simulink model "bh_COMPONENT_car_sys"  (R2018a)
settings: Solver=ode45  StartTime=0.0  StopTime=20  FixedStep=0.001  RelTol=1e-5
undefined symbols (not defined in the file): Ke, mot_bR, mot_COM, veh
libraries: simulink_extras x3, simulink x2
settings Model: Creator=bhorton  LastModifiedBy=bhorton
settings SolverCC: ZeroCrossControl=EnableAll  ZeroCrossAlgorithm=Adaptive
settings DebuggingCC: SignalInfNanChecking=warning
settings ModelReferenceCC: ModelReferenceMinAlgLoopOccurrences=on

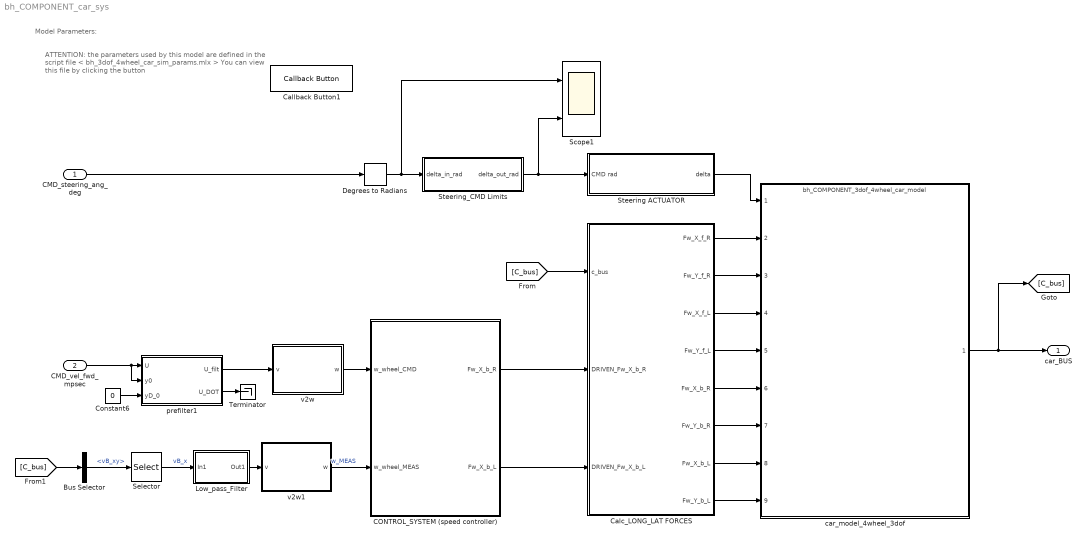
== system bh_COMPONENT_car_sys ==
  note: Model Parameters:
  note: ATTENTION:
      | the parameters used by this model are defined in the script file
      | < bh_3dof_4wheel_car_sim_params.mlx >
      |
      | You can view this file by clicking the button
  CMD_steering_ang_deg : Inport
  CMD_vel_fwd_mpsec : Inport  Port=2
  Bus Selector : BusSelector  OutputSignals=states_B.vB_xy
  CONTROL_SYSTEM (speed controller) : Subsystem  Variant=on  OverrideUsingVariant=Variant1
  Calc_LONG_LAT FORCES : Subsystem
  Callback Button1 : CallbackButton  WebBlockId=2544  ButtonText=view parameter file
      settings: ClickFcn=edit bh_3dof_4wheel_car_sim_params.mlx
  Constant6 : Constant  Value=0
  Degrees to Radians : simulink_extras/Transformations/Degrees to Radians
  Low_pass_Filter : Subsystem
  Scope1 : Scope  NumInputPorts=2
  Selector : Selector  InputPortWidth=2  IndexOptions=Index vector (dialog)  Indices=1  OutputSizes=1
  Steering ACTUATOR : Subsystem
  Steering_CMD Limits : Subsystem
  Terminator : Terminator
  car_model_4wheel_3dof : ModelReference  ModelNameDialog=bh_COMPONENT_3dof_4wheel_car_model.slx  SimulationMode=Normal  ModelReferenceVersion=1.187
  prefilter1 : Subsystem  mask(Derivative Estimation){wn=2*pi*5, p=1}
      mask prompts: wn "Natural frequency, wn (rad/sec)"; p "Damping ratio, p"
      mask help:
      | A simple derivative estimator using a 2nd order representation between input and output.
      |
      | The integrators use a discrete FORWARd Euler rule, and a sample time needs to be specified.
      mask init:
      | str1 = sprintf('wn = %.2f', wn);
      | str2 = sprintf('p  = %.2f', p);
      | %str3 = sprintf('dt = %.2f', dt);
      | %str = char(str1,str2,str3);
      | %str3 = sprintf('dt = %.2f', dt);
      | str = char(str1,str2);
      mask Display: disp(str)
  v2w : Subsystem  mask(v2w){r=veh.wheel.r}
      mask prompts: r "wheel radius (m)"
      mask help:
      | convert v into w
      | w = v/r
      mask Display: image(imread('bh_PIC_v2w.JPG'),'center')
  v2w1 : Subsystem  mask(v2w){r=veh.wheel.r}
      mask prompts: r "wheel radius (m)"
      mask help:
      | convert v into w
      | w = v/r
      mask Display: image(imread('bh_PIC_v2w.JPG'),'center')
  car_BUS : Outport  OutDataTypeStr=Bus: car_BUS
  wires:
  [C_bus] -> Calc_LONG_LAT FORCES/1(c_bus)
  Degrees to Radians/1 -> Scope1/1, Steering_CMD Limits/1(delta_in_rad)
  [C_bus] -> Bus Selector/1
  CMD_vel_fwd_mpsec/1 -> prefilter1/2(y0), prefilter1/1(U)
  Constant6/1 -> prefilter1/3(yD_0)
  CMD_steering_ang_deg/1 -> Degrees to Radians/1
  Steering_CMD Limits/1(delta_out_rad) -> Scope1/2, Steering ACTUATOR/1(CMD rad)
  car_model_4wheel_3dof/1 -> car_BUS/1, [C_bus]
  Steering ACTUATOR/1(delta) -> car_model_4wheel_3dof/1
  Calc_LONG_LAT FORCES/1(Fw_X_f_R) -> car_model_4wheel_3dof/2
  Calc_LONG_LAT FORCES/2(Fw_Y_f_R) -> car_model_4wheel_3dof/3
  Calc_LONG_LAT FORCES/3(Fw_X_f_L) -> car_model_4wheel_3dof/4
  Calc_LONG_LAT FORCES/4(Fw_Y_f_L) -> car_model_4wheel_3dof/5
  Calc_LONG_LAT FORCES/5(Fw_X_b_R) -> car_model_4wheel_3dof/6
  Calc_LONG_LAT FORCES/6(Fw_Y_b_R) -> car_model_4wheel_3dof/7
  Calc_LONG_LAT FORCES/7(Fw_X_b_L) -> car_model_4wheel_3dof/8
  Calc_LONG_LAT FORCES/8(Fw_Y_b_L) -> car_model_4wheel_3dof/9
  prefilter1/1(U_filt) -> v2w/1(v)
  Low_pass_Filter/1(Out1) -> v2w1/1(v)
  v2w/1(w) -> CONTROL_SYSTEM (speed controller)/1(w_wheel_CMD)
  v2w1/1(w) -> CONTROL_SYSTEM (speed controller)/2(w_wheel_MEAS)  "w_MEAS"
  CONTROL_SYSTEM (speed controller)/2(Fw_X_b_L) -> Calc_LONG_LAT FORCES/3(DRIVEN_Fw_X_b_L)
  CONTROL_SYSTEM (speed controller)/1(Fw_X_b_R) -> Calc_LONG_LAT FORCES/2(DRIVEN_Fw_X_b_R)
  Bus Selector/1 -> Selector/1  "<vB_xy>"
  Selector/1 -> Low_pass_Filter/1(In1)  "vB_x"
  prefilter1/2(U_DOT) -> Terminator/1

== system bh_COMPONENT_car_sys/CONTROL_SYSTEM (speed controller) ==
  note: 1) Add Subsystem or Model blocks as valid variant choices.
      | 2) You cannot connect blocks at this level. At simulation, connectivity is automatically
      | determined, based on the active variant and port name matching.
  w_wheel_CMD : Inport
  w_wheel_MEAS : Inport  Port=2
  DC_motor_simple_FRICT : Subsystem  VariantControl=Variant1
  IDEAL_FORCE_ACTUATOR_SYS : Subsystem  VariantControl=Variant3
  Fw_X_b_R : Outport
  Fw_X_b_L : Outport  Port=2

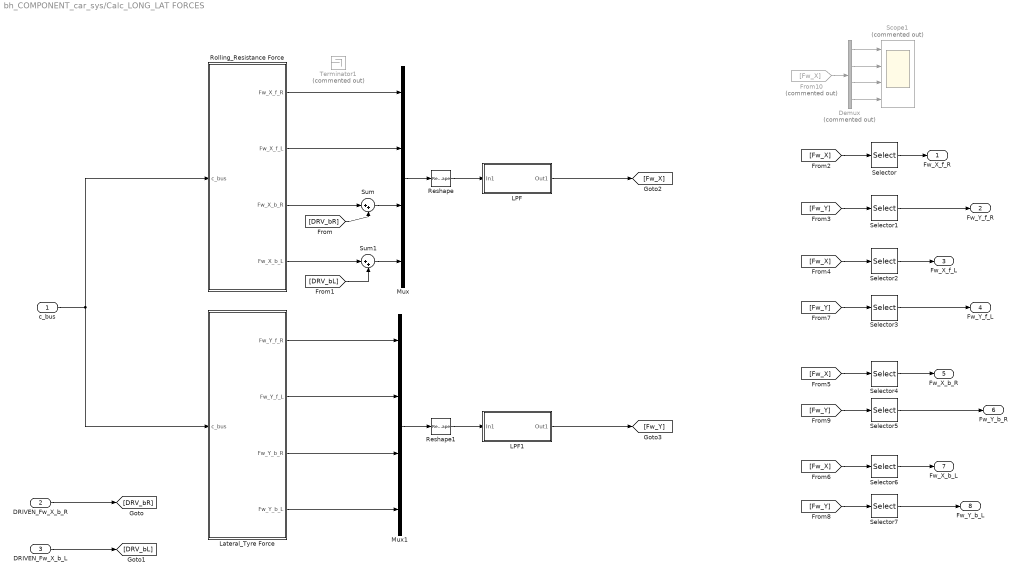
== system bh_COMPONENT_car_sys/Calc_LONG_LAT FORCES ==
  c_bus : Inport
  DRIVEN_Fw_X_b_R : Inport  Port=2
  DRIVEN_Fw_X_b_L : Inport  Port=3
  Demux : Demux  Commented=on
  From10 : From  Commented=on  GotoTag=Fw_X
  LPF : Subsystem
  LPF1 : Subsystem
  Lateral_Tyre Force : Subsystem
  Mux : Mux
  Mux1 : Mux
  Reshape : Reshape  OutputDimensionality=Column vector (2-D)
  Reshape1 : Reshape  OutputDimensionality=Column vector (2-D)
  Rolling_Resistance Force : Subsystem
  Scope1 : Scope  Commented=on  NumInputPorts=4
  Selector : Selector  InputPortWidth=4  IndexOptions=Index vector (dialog)  Indices=1  OutputSizes=1
  Selector1 : Selector  InputPortWidth=4  IndexOptions=Index vector (dialog)  Indices=1  OutputSizes=1
  Selector2 : Selector  InputPortWidth=4  IndexOptions=Index vector (dialog)  Indices=2  OutputSizes=1
  Selector3 : Selector  InputPortWidth=4  IndexOptions=Index vector (dialog)  Indices=2  OutputSizes=1
  Selector4 : Selector  InputPortWidth=4  IndexOptions=Index vector (dialog)  Indices=3  OutputSizes=1
  Selector5 : Selector  InputPortWidth=4  IndexOptions=Index vector (dialog)  Indices=3  OutputSizes=1
  Selector6 : Selector  InputPortWidth=4  IndexOptions=Index vector (dialog)  Indices=4  OutputSizes=1
  Selector7 : Selector  InputPortWidth=4  IndexOptions=Index vector (dialog)  Indices=4  OutputSizes=1
  Sum : Sum  Inputs=|++
  Sum1 : Sum  Inputs=|++
  Terminator1 : Terminator  Commented=on
  Fw_X_f_R : Outport
  Fw_Y_f_R : Outport  Port=2
  Fw_X_f_L : Outport  Port=3
  Fw_Y_f_L : Outport  Port=4
  Fw_X_b_R : Outport  Port=5
  Fw_Y_b_R : Outport  Port=6
  Fw_X_b_L : Outport  Port=7
  Fw_Y_b_L : Outport  Port=8
  wires:
  Selector/1 -> Fw_X_f_R/1
  Selector5/1 -> Fw_Y_b_R/1
  Selector7/1 -> Fw_Y_b_L/1
  Selector1/1 -> Fw_Y_f_R/1
  c_bus/1 -> Rolling_Resistance Force/1(c_bus), Lateral_Tyre Force/1(c_bus)
  DRIVEN_Fw_X_b_R/1 -> [DRV_bR]
  DRIVEN_Fw_X_b_L/1 -> [DRV_bL]
  Rolling_Resistance Force/2(Fw_X_f_L) -> Mux/2
  Rolling_Resistance Force/1(Fw_X_f_R) -> Mux/1
  Lateral_Tyre Force/1(Fw_Y_f_R) -> Mux1/1
  Lateral_Tyre Force/2(Fw_Y_f_L) -> Mux1/2
  Lateral_Tyre Force/3(Fw_Y_b_R) -> Mux1/3
  Lateral_Tyre Force/4(Fw_Y_b_L) -> Mux1/4
  Mux1/1 -> Reshape1/1
  Mux/1 -> Reshape/1
  [Fw_Y] -> Selector1/1
  [Fw_X] -> Selector/1
  Selector6/1 -> Fw_X_b_L/1
  Selector4/1 -> Fw_X_b_R/1
  Selector3/1 -> Fw_Y_f_L/1
  Selector2/1 -> Fw_X_f_L/1
  [Fw_Y] -> Selector7/1
  [Fw_X] -> Selector6/1
  [Fw_Y] -> Selector5/1
  [Fw_X] -> Selector4/1
  [Fw_Y] -> Selector3/1
  [Fw_X] -> Selector2/1
  Reshape/1 -> LPF/1(In1)
  LPF/1(Out1) -> [Fw_X]
  LPF1/1(Out1) -> [Fw_Y]
  Demux/1 -> Scope1/1
  Demux/2 -> Scope1/2
  Demux/3 -> Scope1/3
  Demux/4 -> Scope1/4
  From10/1 -> Demux/1
  Rolling_Resistance Force/3(Fw_X_b_R) -> Sum/1
  [DRV_bR] -> Sum/2
  Sum1/1 -> Mux/4
  Rolling_Resistance Force/4(Fw_X_b_L) -> Sum1/1
  [DRV_bL] -> Sum1/2
  Sum/1 -> Mux/3
  Reshape1/1 -> LPF1/1(In1)

== system bh_COMPONENT_car_sys/Low_pass_Filter ==
  In1 : Inport
  Constant2 : Constant  Value=0
  Terminator1 : Terminator
  prefilter2 : Subsystem  mask(Derivative Estimation){wn=2*pi*100, p=1}
      mask prompts: wn "Natural frequency, wn (rad/sec)"; p "Damping ratio, p"
      mask help:
      | A simple derivative estimator using a 2nd order representation between input and output.
      |
      | The integrators use a discrete FORWARd Euler rule, and a sample time needs to be specified.
      mask init:
      | str1 = sprintf('wn = %.2f', wn);
      | str2 = sprintf('p  = %.2f', p);
      | %str3 = sprintf('dt = %.2f', dt);
      | %str = char(str1,str2,str3);
      | %str3 = sprintf('dt = %.2f', dt);
      | str = char(str1,str2);
      mask Display: disp(str)
  Out1 : Outport
  wires:
  prefilter2/2(U_DOT) -> Terminator1/1
  In1/1 -> prefilter2/1(U)
  prefilter2/1(U_filt) -> Out1/1
  Constant2/1 -> prefilter2/3(yD_0), prefilter2/2(y0)

== system bh_COMPONENT_car_sys/Steering ACTUATOR ==
  CMD rad : Inport
  2nd_order_TF : Subsystem  mask(Derivative Estimation){wn=2*pi*10, p=1}
      mask prompts: wn "Natural frequency, wn (rad/sec)"; p "Damping ratio, p"
      mask help:
      | A simple derivative estimator using a 2nd order representation between input and output.
      |
      | The integrators use a discrete FORWARd Euler rule, and a sample time needs to be specified.
      mask init:
      | str1 = sprintf('wn = %.2f', wn);
      | str2 = sprintf('p  = %.2f', p);
      | %str3 = sprintf('dt = %.2f', dt);
      | %str = char(str1,str2,str3);
      | %str3 = sprintf('dt = %.2f', dt);
      | str = char(str1,str2);
      mask Display: disp(str)
  Constant2 : Constant  Value=0
  Terminator1 : Terminator
  delta : Outport
  wires:
  2nd_order_TF/2(U_DOT) -> Terminator1/1
  CMD rad/1 -> 2nd_order_TF/1(U)
  2nd_order_TF/1(U_filt) -> delta/1
  Constant2/1 -> 2nd_order_TF/3(yD_0), 2nd_order_TF/2(y0)

== system bh_COMPONENT_car_sys/Steering_CMD Limits ==
  note: Saturate on DEGREES
  delta_in_rad : Inport
  Degrees to Radians : simulink_extras/Transformations/Degrees to Radians
  Radians to Degrees : simulink_extras/Transformations/Radians to Degrees
  Saturation : Saturate  UpperLimit=veh.steering_delta_deg_max  LowerLimit=veh.steering_delta_deg_min
      settings: AttributesFormatString=|
      | MAX = %<UpperLimit>
      | MIN = %<LowerLimit>
  delta_out_rad : Outport
  wires:
  delta_in_rad/1 -> Radians to Degrees/1  "radians"
  Saturation/1 -> Degrees to Radians/1  "degrees"
  Radians to Degrees/1 -> Saturation/1  "degrees"
  Degrees to Radians/1 -> delta_out_rad/1  "radians"

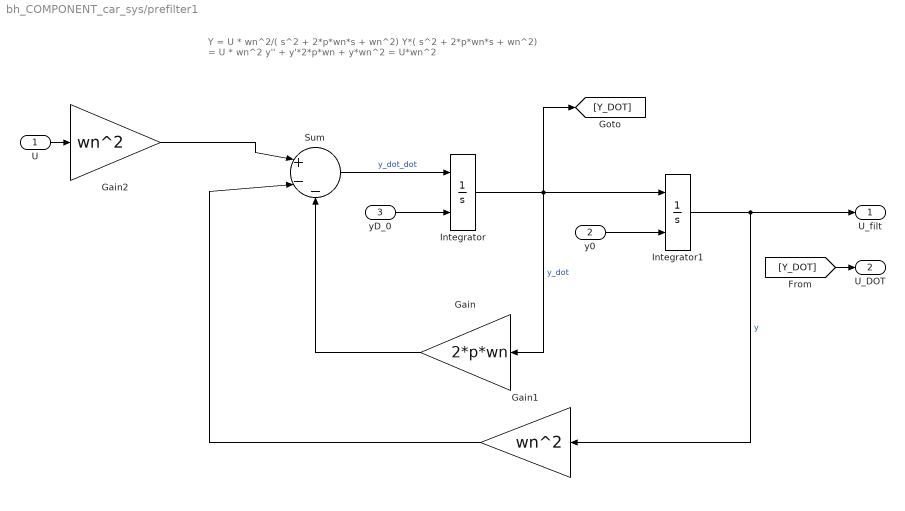
== system bh_COMPONENT_car_sys/prefilter1 ==
  note: Y = U *     wn^2/( s^2 + 2*p*wn*s + wn^2)
      | Y*( s^2 + 2*p*wn*s + wn^2) = U * wn^2
      |
      | y'' + y'*2*p*wn + y*wn^2 = U*wn^2
  U : Inport
  y0 : Inport  Port=2
  yD_0 : Inport  Port=3
  Gain : Gain  Gain=2*p*wn
  Gain1 : Gain  Gain=wn^2
  Gain2 : Gain  Gain=wn^2
  Integrator : Integrator  InitialConditionSource=external
  Integrator1 : Integrator  InitialConditionSource=external
  Sum : Sum  Inputs=|+--
  U_filt : Outport
  U_DOT : Outport  Port=2
  wires:
  Integrator/1 -> [Y_DOT], Gain/1, Integrator1/1  "y_dot"
  Sum/1 -> Integrator/1  "y_dot_dot"
  Integrator1/1 -> Gain1/1, U_filt/1  "y"
  U/1 -> Gain2/1
  Gain2/1 -> Sum/1
  Gain/1 -> Sum/3
  Gain1/1 -> Sum/2
  [Y_DOT] -> U_DOT/1
  yD_0/1 -> Integrator/2
  y0/1 -> Integrator1/2

== system bh_COMPONENT_car_sys/v2w ==
  note: w = v/r
  v : Inport
  Gain : Gain  Gain=1/r
  w : Outport
  wires:
  v/1 -> Gain/1
  Gain/1 -> w/1

== system bh_COMPONENT_car_sys/v2w1 ==
  note: w = v/r
  v : Inport
  Gain : Gain  Gain=1/r
  w : Outport
  wires:
  v/1 -> Gain/1
  Gain/1 -> w/1

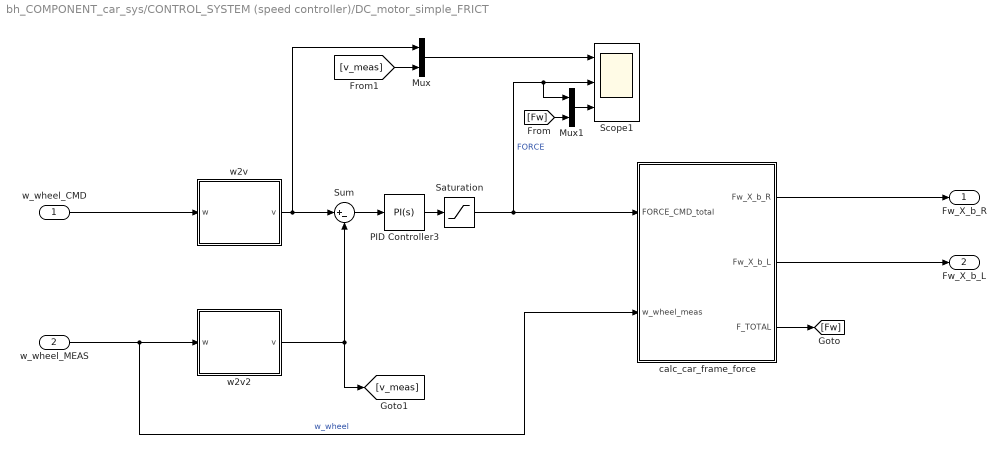
== system bh_COMPONENT_car_sys/CONTROL_SYSTEM (speed controller)/DC_motor_simple_FRICT ==
  w_wheel_CMD : Inport
  w_wheel_MEAS : Inport  Port=2
  Mux : Mux  Inputs=2
  Mux1 : Mux  Inputs=2
  PID Controller3 : simulink/Continuous/PID Controller  Controller=PI  TimeDomain=Continuous-time  SampleTime=-1  IntegratorMethod=Forward Euler  FilterMethod=Forward Euler  Form=Parallel  UseFilter=on  ControllerParametersSource=internal  P=7.09625612003908  I=0.587579927612706  D=0  N=100  InitialConditionSource=internal  InitialConditionForIntegrator=0  InitialConditionForFilter=0  ExternalReset=none  LimitOutput=off  UpperSaturationLimit=inf  LowerSaturationLimit=-inf  LinearizeAsGain=on  AntiWindupMode=none  Kb=1  TrackingMode=off  Kt=1  PParamMin=[]  PParamMax=[]  IParamMin=[]  IParamMax=[]  DParamMin=[]  DParamMax=[]  NParamMin=[]  NParamMax=[]  KbParamMin=[]  KbParamMax=[]  KtParamMin=[]  KtParamMax=[]  POutMin=[]  POutMax=[]  IOutMin=[]  IOutMax=[]  DOutMin=[]  DOutMax=[]  NOutMin=[]  NOutMax=[]  KbOutMin=[]  KbOutMax=[]  KtOutMin=[]  KtOutMax=[]  IntegratorOutMin=[]  IntegratorOutMax=[]  FilterOutMin=[]  FilterOutMax=[]  SumOutMin=[]  SumOutMax=[]  SumI1OutMin=[]  SumI1OutMax=[]  SumI2OutMin=[]  SumI2OutMax=[]  SumI3OutMin=[]  SumI3OutMax=[]  SumDOutMin=[]  SumDOutMax=[]  SaturationOutMin=[]  SaturationOutMax=[]  IntegratorContinuousStateAttributes=''  IntegratorStateMustResolveToSignalObject=off  IntegratorRTWStateStorageClass=Auto  FilterContinuousStateAttributes=''  FilterStateMustResolveToSignalObject=off  FilterRTWStateStorageClass=Auto  DifferentiatorICPrevScaledInput=0  DifferentiatorOutMin=[]  DifferentiatorOutMax=[]  InitialConditionSetting=State (most efficient)  FilterDiffOutCoefMin=[]  FilterDiffOutCoefMax=[]  SumDenOutMin=[]  SumDenOutMax=[]  SumNumOutMin=[]  SumNumOutMax=[]  ReciprocalOutMin=[]  ReciprocalOutMax=[]  DivideOutMin=[]  DivideOutMax=[]  TunerSelectOption=Transfer Function Based (PID Tuner App)
  Saturation : Saturate  UpperLimit=1  LowerLimit=-1
      settings: AttributesFormatString=|
      | Fmax= %<UpperLimit>
      | Fmin= %<LowerLimit>
  Scope1 : Scope  NumInputPorts=3
  Sum : Sum  Inputs=|+-
  calc_car_frame_force : Subsystem
  w2v : Subsystem  mask{r=veh.wheel.r}
      mask prompts: r "wheel radius (m)"
      mask Display: image(imread('bh_PIC_w2v.JPG'),'center')
  w2v2 : Subsystem  mask{r=veh.wheel.r}
      mask prompts: r "wheel radius (m)"
      mask Display: image(imread('bh_PIC_w2v.JPG'),'center')
  Fw_X_b_R : Outport
  Fw_X_b_L : Outport  Port=2
  wires:
  w2v/1(v) -> Mux/1, Sum/1
  [v_meas] -> Mux/2
  Saturation/1 -> calc_car_frame_force/1(FORCE_CMD_total), Mux1/1, Scope1/2  "FORCE"
  Sum/1 -> PID Controller3/1
  Mux/1 -> Scope1/1
  w_wheel_CMD/1 -> w2v/1(w)
  PID Controller3/1 -> Saturation/1
  w2v2/1(v) -> [v_meas], Sum/2
  w_wheel_MEAS/1 -> calc_car_frame_force/2(w_wheel_meas), w2v2/1(w)  "w_wheel"
  Mux1/1 -> Scope1/3
  [Fw] -> Mux1/2
  calc_car_frame_force/2(Fw_X_b_L) -> Fw_X_b_L/1
  calc_car_frame_force/1(Fw_X_b_R) -> Fw_X_b_R/1
  calc_car_frame_force/3(F_TOTAL) -> [Fw]

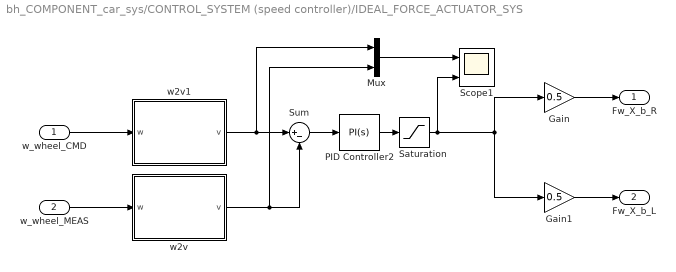
== system bh_COMPONENT_car_sys/CONTROL_SYSTEM (speed controller)/IDEAL_FORCE_ACTUATOR_SYS ==
  w_wheel_CMD : Inport
  w_wheel_MEAS : Inport  Port=2
  Gain : Gain  Gain=0.5
  Gain1 : Gain  Gain=0.5
  Mux : Mux  Inputs=2
  PID Controller2 : simulink/Continuous/PID Controller  Controller=PI  TimeDomain=Continuous-time  SampleTime=-1  IntegratorMethod=Forward Euler  FilterMethod=Forward Euler  Form=Parallel  UseFilter=on  ControllerParametersSource=internal  P=7.09625612003908  I=0.587579927612706  D=0  N=100  InitialConditionSource=internal  InitialConditionForIntegrator=0  InitialConditionForFilter=0  ExternalReset=none  LimitOutput=off  UpperSaturationLimit=inf  LowerSaturationLimit=-inf  LinearizeAsGain=on  AntiWindupMode=none  Kb=1  TrackingMode=off  Kt=1  PParamMin=[]  PParamMax=[]  IParamMin=[]  IParamMax=[]  DParamMin=[]  DParamMax=[]  NParamMin=[]  NParamMax=[]  KbParamMin=[]  KbParamMax=[]  KtParamMin=[]  KtParamMax=[]  POutMin=[]  POutMax=[]  IOutMin=[]  IOutMax=[]  DOutMin=[]  DOutMax=[]  NOutMin=[]  NOutMax=[]  KbOutMin=[]  KbOutMax=[]  KtOutMin=[]  KtOutMax=[]  IntegratorOutMin=[]  IntegratorOutMax=[]  FilterOutMin=[]  FilterOutMax=[]  SumOutMin=[]  SumOutMax=[]  SumI1OutMin=[]  SumI1OutMax=[]  SumI2OutMin=[]  SumI2OutMax=[]  SumI3OutMin=[]  SumI3OutMax=[]  SumDOutMin=[]  SumDOutMax=[]  SaturationOutMin=[]  SaturationOutMax=[]  IntegratorContinuousStateAttributes=''  IntegratorStateMustResolveToSignalObject=off  IntegratorRTWStateStorageClass=Auto  FilterContinuousStateAttributes=''  FilterStateMustResolveToSignalObject=off  FilterRTWStateStorageClass=Auto  DifferentiatorICPrevScaledInput=0  DifferentiatorOutMin=[]  DifferentiatorOutMax=[]  InitialConditionSetting=State (most efficient)  FilterDiffOutCoefMin=[]  FilterDiffOutCoefMax=[]  SumDenOutMin=[]  SumDenOutMax=[]  SumNumOutMin=[]  SumNumOutMax=[]  ReciprocalOutMin=[]  ReciprocalOutMax=[]  DivideOutMin=[]  DivideOutMax=[]  TunerSelectOption=Transfer Function Based (PID Tuner App)
  Saturation : Saturate  UpperLimit=1  LowerLimit=-1
  Scope1 : Scope  NumInputPorts=2
  Sum : Sum  Inputs=|+-
  w2v : Subsystem  mask(w2v){r=veh.wheel.r}
      mask prompts: r "wheel radius (m)"
      mask help:
      | convert w into v
      | v = w * r
      mask Display: image(imread('bh_PIC_w2v.JPG'),'center')
  w2v1 : Subsystem  mask(w2v){r=veh.wheel.r}
      mask prompts: r "wheel radius (m)"
      mask help:
      | convert w into v
      | v = w * r
      mask Display: image(imread('bh_PIC_w2v.JPG'),'center')
  Fw_X_b_R : Outport
  Fw_X_b_L : Outport  Port=2
  wires:
  Saturation/1 -> Scope1/2, Gain1/1, Gain/1
  PID Controller2/1 -> Saturation/1
  Gain1/1 -> Fw_X_b_L/1
  Gain/1 -> Fw_X_b_R/1
  w_wheel_CMD/1 -> w2v1/1(w)
  Sum/1 -> PID Controller2/1
  w_wheel_MEAS/1 -> w2v/1(w)
  Mux/1 -> Scope1/1
  w2v1/1(v) -> Mux/1, Sum/1
  w2v/1(v) -> Mux/2, Sum/2

== system bh_COMPONENT_car_sys/Calc_LONG_LAT FORCES/LPF ==
  In1 : Inport
  Constant2 : Constant  Value=[0;0;0;0]  VectorParams1D=off
  Terminator1 : Terminator
  prefilter2 : Subsystem  mask(Derivative Estimation){wn=2*pi*100, p=1}
      mask prompts: wn "Natural frequency, wn (rad/sec)"; p "Damping ratio, p"
      mask help:
      | A simple derivative estimator using a 2nd order representation between input and output.
      |
      | The integrators use a discrete FORWARd Euler rule, and a sample time needs to be specified.
      mask init:
      | str1 = sprintf('wn = %.2f', wn);
      | str2 = sprintf('p  = %.2f', p);
      | %str3 = sprintf('dt = %.2f', dt);
      | %str = char(str1,str2,str3);
      | %str3 = sprintf('dt = %.2f', dt);
      | str = char(str1,str2);
      mask Display: disp(str)
  Out1 : Outport
  wires:
  prefilter2/2(U_DOT) -> Terminator1/1
  Constant2/1 -> prefilter2/2(y0), prefilter2/3(yD_0)
  prefilter2/1(U_filt) -> Out1/1
  In1/1 -> prefilter2/1(U)

== system bh_COMPONENT_car_sys/Calc_LONG_LAT FORCES/LPF1 ==
  In1 : Inport
  Constant2 : Constant  Value=[0;0;0;0]  VectorParams1D=off
  Terminator1 : Terminator
  prefilter2 : Subsystem  mask(Derivative Estimation){wn=2*pi*100, p=1}
      mask prompts: wn "Natural frequency, wn (rad/sec)"; p "Damping ratio, p"
      mask help:
      | A simple derivative estimator using a 2nd order representation between input and output.
      |
      | The integrators use a discrete FORWARd Euler rule, and a sample time needs to be specified.
      mask init:
      | str1 = sprintf('wn = %.2f', wn);
      | str2 = sprintf('p  = %.2f', p);
      | %str3 = sprintf('dt = %.2f', dt);
      | %str = char(str1,str2,str3);
      | %str3 = sprintf('dt = %.2f', dt);
      | str = char(str1,str2);
      mask Display: disp(str)
  Out1 : Outport
  wires:
  prefilter2/2(U_DOT) -> Terminator1/1
  Constant2/1 -> prefilter2/2(y0), prefilter2/3(yD_0)
  prefilter2/1(U_filt) -> Out1/1
  In1/1 -> prefilter2/1(U)

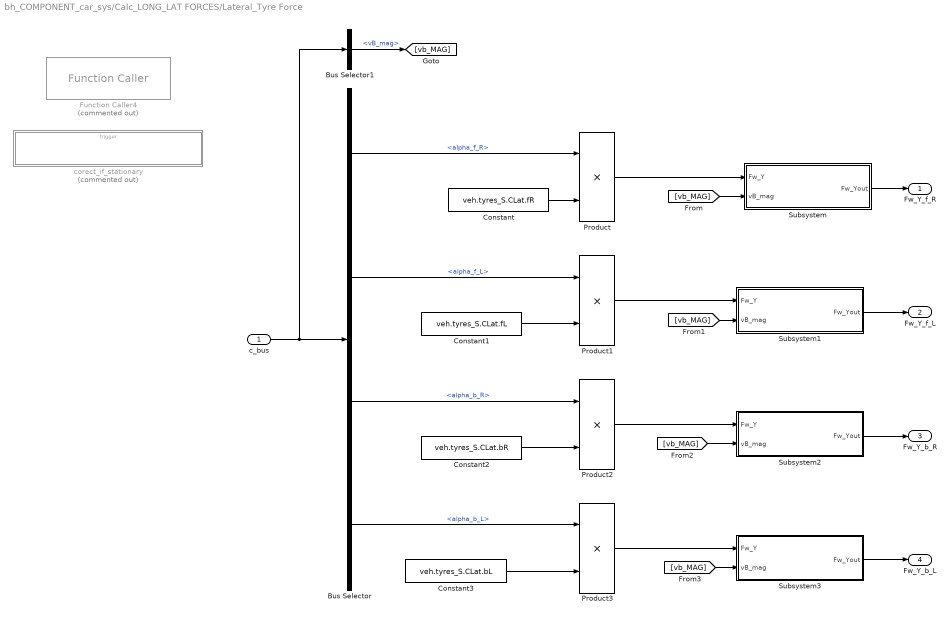
== system bh_COMPONENT_car_sys/Calc_LONG_LAT FORCES/Lateral_Tyre Force ==
  c_bus : Inport
  Bus Selector : BusSelector  OutputSignals=alpha.alpha_f_R,alpha.alpha_f_L,alpha.alpha_b_R,alpha.alpha_b_L
  Bus Selector1 : BusSelector  OutputSignals=states_B.vB_mag
  Constant : Constant  Value=veh.tyres_S.CLat.fR
  Constant1 : Constant  Value=veh.tyres_S.CLat.fL
  Constant2 : Constant  Value=veh.tyres_S.CLat.bR
  Constant3 : Constant  Value=veh.tyres_S.CLat.bL
  Function Caller4 : FunctionCaller  Commented=on  FunctionPrototype=y = correct_if_stationary(Fw_Y,vb_MAG)  InputArgumentSpecifications=double(1), double(1)  OutputArgumentSpecifications=double(1)
  Product{,1..3} (4 alike) : Product
  Subsystem : Subsystem
  Subsystem1 : Subsystem
  Subsystem2 : Subsystem
  Subsystem3 : Subsystem
  corect_if_stationary : Subsystem  Commented=on  TreatAsAtomicUnit=on
  Fw_Y_f_R : Outport
  Fw_Y_f_L : Outport  Port=2
  Fw_Y_b_R : Outport  Port=3
  Fw_Y_b_L : Outport  Port=4
  wires:
  c_bus/1 -> Bus Selector1/1, Bus Selector/1
  Bus Selector/1 -> Product/1  "<alpha_f_R>"
  Constant/1 -> Product/2
  Bus Selector/2 -> Product1/1  "<alpha_f_L>"
  Constant1/1 -> Product1/2
  Bus Selector/3 -> Product2/1  "<alpha_b_R>"
  Constant2/1 -> Product2/2
  Bus Selector/4 -> Product3/1  "<alpha_b_L>"
  Constant3/1 -> Product3/2
  Bus Selector1/1 -> [vb_MAG]  "<vB_mag>"
  Product/1 -> Subsystem/1(Fw_Y)
  Subsystem/1(Fw_Yout) -> Fw_Y_f_R/1
  Subsystem1/1(Fw_Yout) -> Fw_Y_f_L/1
  Subsystem2/1(Fw_Yout) -> Fw_Y_b_R/1
  Subsystem3/1(Fw_Yout) -> Fw_Y_b_L/1
  [vb_MAG] -> Subsystem/2(vB_mag)
  Product1/1 -> Subsystem1/1(Fw_Y)
  Product2/1 -> Subsystem2/1(Fw_Y)
  Product3/1 -> Subsystem3/1(Fw_Y)
  [vb_MAG] -> Subsystem1/2(vB_mag)
  [vb_MAG] -> Subsystem2/2(vB_mag)
  [vb_MAG] -> Subsystem3/2(vB_mag)

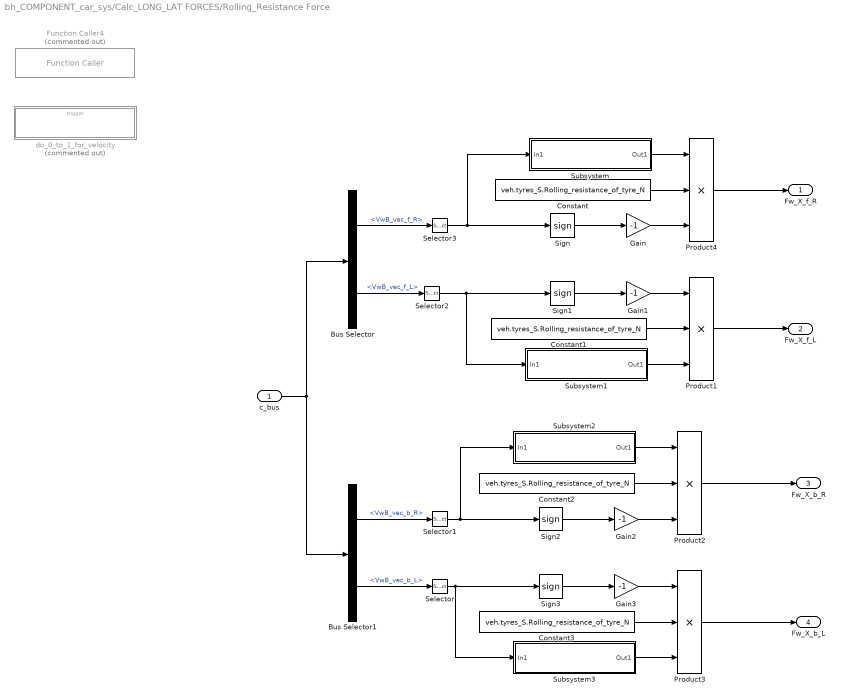
== system bh_COMPONENT_car_sys/Calc_LONG_LAT FORCES/Rolling_Resistance Force ==
  c_bus : Inport
  Bus Selector : BusSelector  OutputSignals=wheel.VwB_vec_f_R,wheel.VwB_vec_f_L
  Bus Selector1 : BusSelector  OutputSignals=wheel.VwB_vec_b_R,wheel.VwB_vec_b_L
  Constant{,1..3} (4 alike) : Constant  Value=veh.tyres_S.Rolling_resistance_of_tyre_N
  Function Caller4 : FunctionCaller  Commented=on  FunctionPrototype=y = zero_to_1_from_VEL(u)  InputArgumentSpecifications=double(1)  OutputArgumentSpecifications=double(1)
  Gain{,1..3} (4 alike) : Gain  Gain=-1
  Product{1..4} (4 alike) : Product  Inputs=3
  Selector{,1..3} (4 alike) : Selector  InputPortWidth=2  IndexOptions=Index vector (dialog)  Indices=1  OutputSizes=1
  Sign{,1..3} (4 alike) : Signum
  Subsystem : Subsystem
  Subsystem1 : Subsystem
  Subsystem2 : Subsystem
  Subsystem3 : Subsystem
  do_0_to_1_for_velocity : Subsystem  Commented=on  TreatAsAtomicUnit=on
  Fw_X_f_R : Outport
  Fw_X_f_L : Outport  Port=2
  Fw_X_b_R : Outport  Port=3
  Fw_X_b_L : Outport  Port=4
  wires:
  c_bus/1 -> Bus Selector1/1, Bus Selector/1
  Bus Selector/1 -> Selector3/1  "<VwB_vec_f_R>"
  Bus Selector/2 -> Selector2/1  "<VwB_vec_f_L>"
  Sign/1 -> Gain/1
  Sign1/1 -> Gain1/1
  Gain/1 -> Product4/3
  Gain1/1 -> Product1/1
  Constant/1 -> Product4/2
  Constant1/1 -> Product1/2
  Product1/1 -> Fw_X_f_L/1
  Product4/1 -> Fw_X_f_R/1
  Gain2/1 -> Product2/3
  Sign3/1 -> Gain3/1
  Gain3/1 -> Product3/1
  Bus Selector1/1 -> Selector1/1  "<VwB_vec_b_R>"
  Constant2/1 -> Product2/2
  Sign2/1 -> Gain2/1
  Product3/1 -> Fw_X_b_L/1
  Product2/1 -> Fw_X_b_R/1
  Constant3/1 -> Product3/2
  Bus Selector1/2 -> Selector/1  "<VwB_vec_b_L>"
  Subsystem1/1(Out1) -> Product1/3
  Subsystem/1(Out1) -> Product4/1
  Subsystem2/1(Out1) -> Product2/1
  Subsystem3/1(Out1) -> Product3/3
  Selector3/1 -> Subsystem/1(In1), Sign/1
  Selector2/1 -> Subsystem1/1(In1), Sign1/1
  Selector1/1 -> Subsystem2/1(In1), Sign2/1
  Selector/1 -> Subsystem3/1(In1), Sign3/1

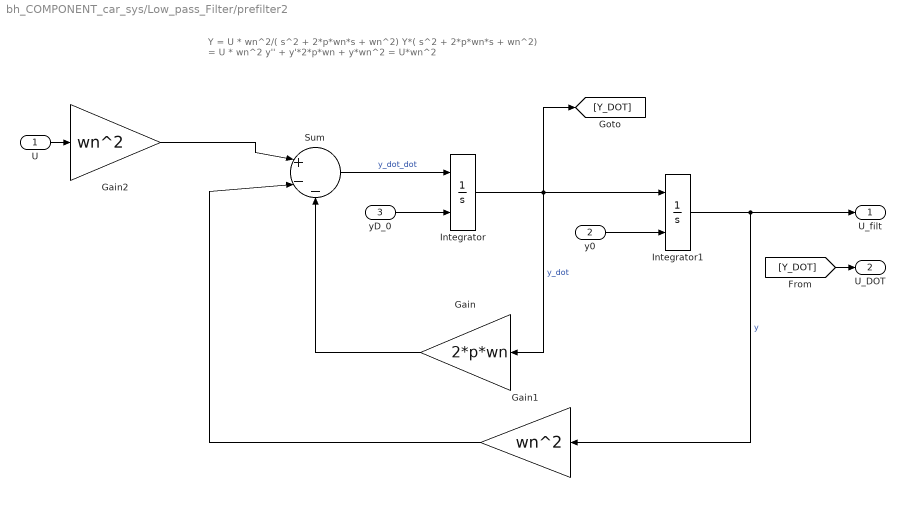
== system bh_COMPONENT_car_sys/Low_pass_Filter/prefilter2 ==
  note: Y = U *     wn^2/( s^2 + 2*p*wn*s + wn^2)
      | Y*( s^2 + 2*p*wn*s + wn^2) = U * wn^2
      |
      | y'' + y'*2*p*wn + y*wn^2 = U*wn^2
  U : Inport
  y0 : Inport  Port=2
  yD_0 : Inport  Port=3
  Gain : Gain  Gain=2*p*wn
  Gain1 : Gain  Gain=wn^2
  Gain2 : Gain  Gain=wn^2
  Integrator : Integrator  InitialConditionSource=external
  Integrator1 : Integrator  InitialConditionSource=external
  Sum : Sum  Inputs=|+--
  U_filt : Outport
  U_DOT : Outport  Port=2
  wires:
  Integrator/1 -> [Y_DOT], Gain/1, Integrator1/1  "y_dot"
  Sum/1 -> Integrator/1  "y_dot_dot"
  Integrator1/1 -> Gain1/1, U_filt/1  "y"
  U/1 -> Gain2/1
  Gain2/1 -> Sum/1
  Gain/1 -> Sum/3
  Gain1/1 -> Sum/2
  [Y_DOT] -> U_DOT/1
  yD_0/1 -> Integrator/2
  y0/1 -> Integrator1/2

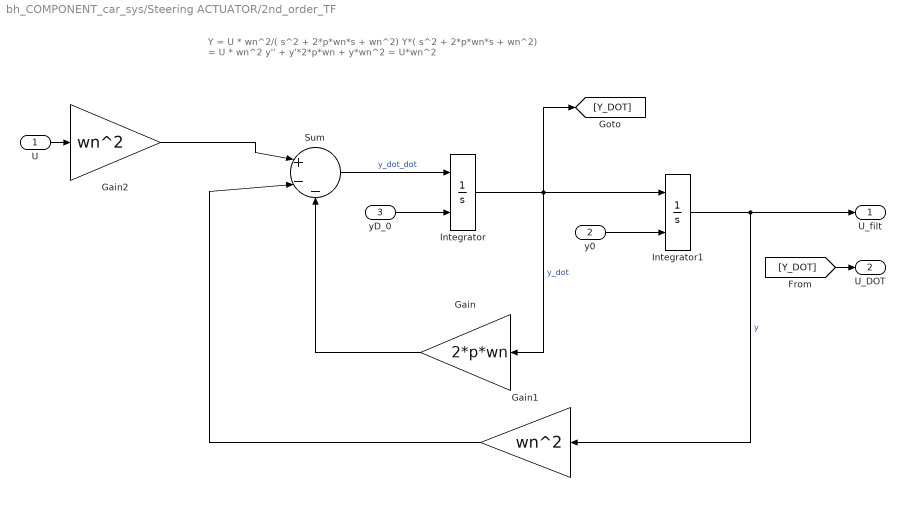
== system bh_COMPONENT_car_sys/Steering ACTUATOR/2nd_order_TF ==
  note: Y = U *     wn^2/( s^2 + 2*p*wn*s + wn^2)
      | Y*( s^2 + 2*p*wn*s + wn^2) = U * wn^2
      |
      | y'' + y'*2*p*wn + y*wn^2 = U*wn^2
  U : Inport
  y0 : Inport  Port=2
  yD_0 : Inport  Port=3
  Gain : Gain  Gain=2*p*wn
  Gain1 : Gain  Gain=wn^2
  Gain2 : Gain  Gain=wn^2
  Integrator : Integrator  InitialConditionSource=external
  Integrator1 : Integrator  InitialConditionSource=external
  Sum : Sum  Inputs=|+--
  U_filt : Outport
  U_DOT : Outport  Port=2
  wires:
  Integrator/1 -> [Y_DOT], Gain/1, Integrator1/1  "y_dot"
  Sum/1 -> Integrator/1  "y_dot_dot"
  Integrator1/1 -> Gain1/1, U_filt/1  "y"
  U/1 -> Gain2/1
  Gain2/1 -> Sum/1
  Gain/1 -> Sum/3
  Gain1/1 -> Sum/2
  [Y_DOT] -> U_DOT/1
  yD_0/1 -> Integrator/2
  y0/1 -> Integrator1/2

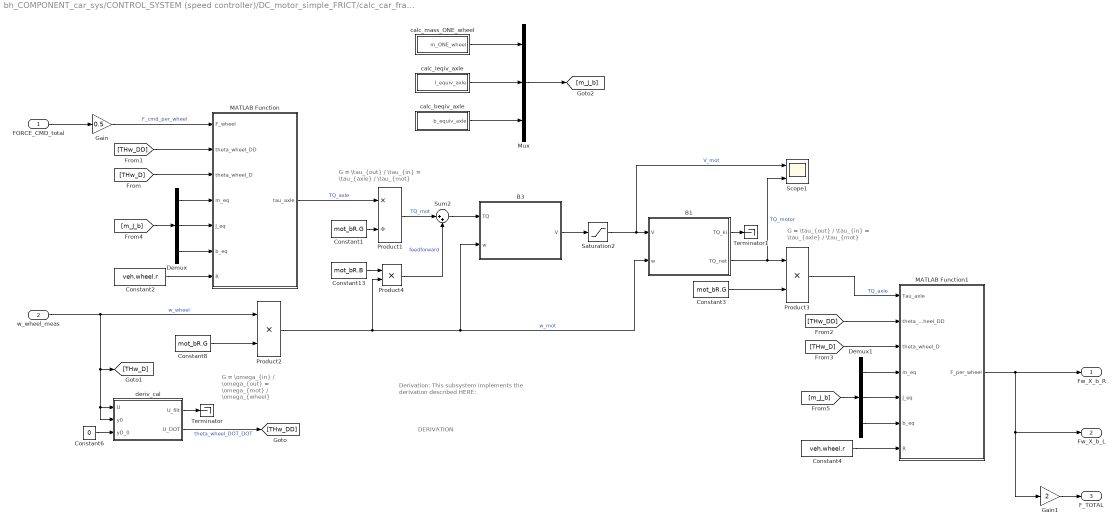
== system bh_COMPONENT_car_sys/CONTROL_SYSTEM (speed controller)/DC_motor_simple_FRICT/calc_car_frame_force ==
  note: DERIVATION
  note: Derivation:
      |
      | This subsystem implements the
      | derivation described HERE:
  note: G = \tau_{out} / \tau_{in} = \tau_{axle} / \tau_{mot}
  note: G = \omega_{in} / \omega_{out} = \omega_{mot} / \omega_{wheel}
  note: G = \tau_{out} / \tau_{in} = \tau_{axle} / \tau_{mot}
  FORCE_CMD_total : Inport
  w_wheel_meas : Inport  Port=2
  B1 : Subsystem  mask(DC motor (w_IN and TQ_out)){R=mot_bR.R, K=mot_bR.K, Kb=Ke, b=mot_bR.B}
      mask prompts: R "Armature resistance (ohms)"; K "Torque constant (N.m/A)"; Kb "Back Emf constant (V.sec/rad)"; b "Viscous friction co-eff (N.m.sec/rad)"
      mask help: A DC motor model that outputs TORQUE for a given speed input
      mask DialogControl Control2 Prompt: NOTE:  with SI units, the Toque constant (Ka) and Back EMF constant(Kb) are the same.
      mask DialogControl Container9 Prompt: Electrical
      mask Display: fprintf('DC motor\n(w_IN \n and \n TQ_out)');
  B3 : Subsystem  mask(DC motor (w_IN and TQ_out)){R=mot_bR.R, K=mot_bR.K, Kb=Ke}
      mask prompts: R "Armature resistance (ohms)"; K "Torque constant (N.m/A)"; Kb "Back Emf constant (V.sec/rad)"
      mask help: A DC motor model that outputs TORQUE for a given speed input
      mask DialogControl Control2 Prompt: NOTE:  with SI units, the Toque constant (Ka) and Back EMF constant(Kb) are the same.
      mask DialogControl Container9 Prompt: Electrical
      mask Display: fprintf('DC motor\n(TQ_IN \n and \n V_out)');
  Constant1 : Constant  Value=mot_bR.G
  Constant13 : Constant  Value=mot_bR.B
  Constant2 : Constant  Value=veh.wheel.r
  Constant3 : Constant  Value=mot_bR.G
  Constant4 : Constant  Value=veh.wheel.r
  Constant6 : Constant  Value=0
  Constant8 : Constant  Value=mot_bR.G
  Demux : Demux  Outputs=3
  Demux1 : Demux  Outputs=3
  Gain : Gain  Gain=0.5
  Gain1 : Gain  Gain=2
  MATLAB Function : MATLAB Function  TreatAsAtomicUnit=on
  MATLAB Function1 : MATLAB Function  TreatAsAtomicUnit=on
  Mux : Mux  Inputs=3
  Product1 : Product  Inputs=*/
  Product2 : Product
  Product3 : Product
  Product4 : Product
  Saturation2 : Saturate  UpperLimit=mot_COM.Vmax_sat  LowerLimit=mot_COM.Vmin_sat
      settings: AttributesFormatString=|
      | %<UpperLimit>
      | %<LowerLimit>
  Scope1 : Scope  NumInputPorts=2
  Sum2 : Sum  Inputs=|++
  Terminator : Terminator
  Terminator1 : Terminator
  calc_Ieqiv_axle : Subsystem
  calc_beqiv_axle : Subsystem
  calc_mass_ONE_wheel : Subsystem
  deriv_cal : Subsystem  mask(Derivative Estimation){wn=2*pi*100, p=1}
      mask prompts: wn "Natural frequency, wn (rad/sec)"; p "Damping ratio, p"
      mask help:
      | A simple derivative estimator using a 2nd order representation between input and output.
      |
      | The integrators use a discrete FORWARd Euler rule, and a sample time needs to be specified.
      mask init:
      | str1 = sprintf('wn = %.2f', wn);
      | str2 = sprintf('p  = %.2f', p);
      | %str3 = sprintf('dt = %.2f', dt);
      | %str = char(str1,str2,str3);
      | %str3 = sprintf('dt = %.2f', dt);
      | str = char(str1,str2);
      mask Display: disp(str)
  Fw_X_b_R : Outport
  Fw_X_b_L : Outport  Port=2
  F_TOTAL : Outport  Port=3
  wires:
  FORCE_CMD_total/1 -> Gain/1
  Constant3/1 -> Product3/2
  Constant1/1 -> Product1/2
  MATLAB Function/1(tau_axle) -> Product1/1  "TQ_axle"
  B3/1(V) -> Saturation2/1
  Saturation2/1 -> B1/1(V), Scope1/1  "V_mot"
  Constant6/1 -> deriv_cal/3(yD_0)
  deriv_cal/1(U_filt) -> Terminator/1
  deriv_cal/2(U_DOT) -> [THw_DD]  "theta_wheel_DOT_DOT"
  Constant8/1 -> Product2/2
  w_wheel_meas/1 -> [THw_D], deriv_cal/1(U), deriv_cal/2(y0), Product2/1  "w_wheel"
  Product2/1 -> Product4/2, B1/2(w), B3/2(w)  "w_mot"
  Product3/1 -> MATLAB Function1/1(Tau_axle)  "TQ_axle"
  B1/2(TQ_net) -> Product3/1, Scope1/2  "TQ_motor"
  Sum2/1 -> B3/1(TQ)
  Product1/1 -> Sum2/1  "TQ_mot"
  Constant13/1 -> Product4/1
  B1/1(TQ_ki) -> Terminator1/1
  [THw_DD] -> MATLAB Function/2(theta_wheel_DD)
  Constant2/1 -> MATLAB Function/7(R)
  Gain/1 -> MATLAB Function/1(F_wheel)  "F_cmd_per_wheel"
  Product4/1 -> Sum2/2  "feedforward"
  MATLAB Function1/1(F_per_wheel) -> Fw_X_b_R/1, Fw_X_b_L/1, Gain1/1
  [THw_DD] -> MATLAB Function1/2(theta_wheel_DD)
  [THw_D] -> MATLAB Function/3(theta_wheel_D)
  [THw_D] -> MATLAB Function1/3(theta_wheel_D)
  calc_beqiv_axle/1(b_equiv_axle) -> Mux/3
  calc_Ieqiv_axle/1(I_equiv_axle) -> Mux/2
  calc_mass_ONE_wheel/1(m_ONE_wheel) -> Mux/1
  Mux/1 -> [m_J_b]
  Demux/1 -> MATLAB Function/4(m_eq)
  Demux/2 -> MATLAB Function/5(J_eq)
  Demux/3 -> MATLAB Function/6(b_eq)
  [m_J_b] -> Demux/1
  Demux1/1 -> MATLAB Function1/4(m_eq)
  Demux1/2 -> MATLAB Function1/5(J_eq)
  Demux1/3 -> MATLAB Function1/6(b_eq)
  [m_J_b] -> Demux1/1
  Constant4/1 -> MATLAB Function1/7(R)
  Gain1/1 -> F_TOTAL/1

== system bh_COMPONENT_car_sys/CONTROL_SYSTEM (speed controller)/DC_motor_simple_FRICT/w2v ==
  note: v = w * r
  w : Inport
  Gain : Gain  Gain=r
  v : Outport
  wires:
  w/1 -> Gain/1
  Gain/1 -> v/1

== system bh_COMPONENT_car_sys/CONTROL_SYSTEM (speed controller)/DC_motor_simple_FRICT/w2v2 ==
  note: v = w * r
  w : Inport
  Gain : Gain  Gain=r
  v : Outport
  wires:
  w/1 -> Gain/1
  Gain/1 -> v/1

== system bh_COMPONENT_car_sys/CONTROL_SYSTEM (speed controller)/IDEAL_FORCE_ACTUATOR_SYS/w2v ==
  note: v = w * r
  w : Inport
  Gain : Gain  Gain=r
  v : Outport
  wires:
  w/1 -> Gain/1
  Gain/1 -> v/1

== system bh_COMPONENT_car_sys/CONTROL_SYSTEM (speed controller)/IDEAL_FORCE_ACTUATOR_SYS/w2v1 ==
  note: v = w * r
  w : Inport
  Gain : Gain  Gain=r
  v : Outport
  wires:
  w/1 -> Gain/1
  Gain/1 -> v/1

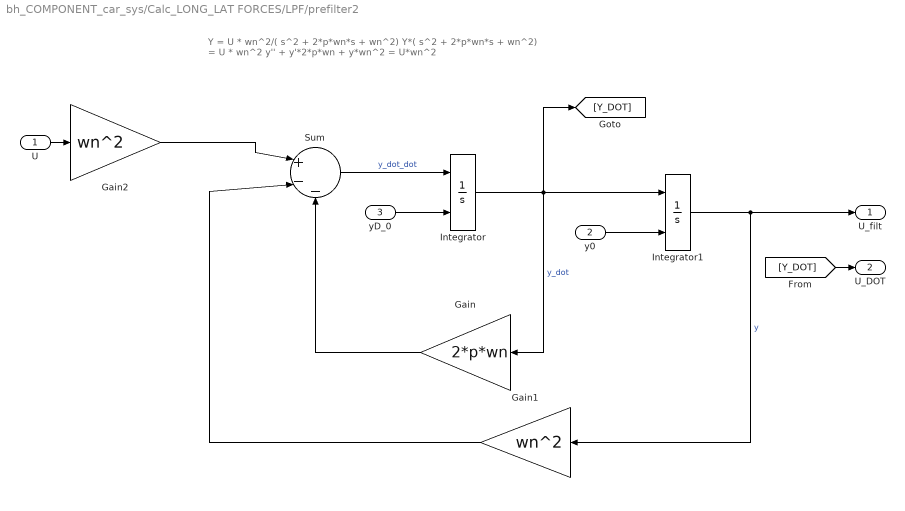
== system bh_COMPONENT_car_sys/Calc_LONG_LAT FORCES/LPF/prefilter2 ==
  note: Y = U *     wn^2/( s^2 + 2*p*wn*s + wn^2)
      | Y*( s^2 + 2*p*wn*s + wn^2) = U * wn^2
      |
      | y'' + y'*2*p*wn + y*wn^2 = U*wn^2
  U : Inport
  y0 : Inport  Port=2
  yD_0 : Inport  Port=3
  Gain : Gain  Gain=2*p*wn
  Gain1 : Gain  Gain=wn^2
  Gain2 : Gain  Gain=wn^2
  Integrator : Integrator  InitialConditionSource=external
  Integrator1 : Integrator  InitialConditionSource=external
  Sum : Sum  Inputs=|+--
  U_filt : Outport
  U_DOT : Outport  Port=2
  wires:
  Integrator/1 -> [Y_DOT], Gain/1, Integrator1/1  "y_dot"
  Sum/1 -> Integrator/1  "y_dot_dot"
  Integrator1/1 -> Gain1/1, U_filt/1  "y"
  U/1 -> Gain2/1
  Gain2/1 -> Sum/1
  Gain/1 -> Sum/3
  Gain1/1 -> Sum/2
  [Y_DOT] -> U_DOT/1
  yD_0/1 -> Integrator/2
  y0/1 -> Integrator1/2

== system bh_COMPONENT_car_sys/Calc_LONG_LAT FORCES/LPF1/prefilter2 ==
  note: Y = U *     wn^2/( s^2 + 2*p*wn*s + wn^2)
      | Y*( s^2 + 2*p*wn*s + wn^2) = U * wn^2
      |
      | y'' + y'*2*p*wn + y*wn^2 = U*wn^2
  U : Inport
  y0 : Inport  Port=2
  yD_0 : Inport  Port=3
  Gain : Gain  Gain=2*p*wn
  Gain1 : Gain  Gain=wn^2
  Gain2 : Gain  Gain=wn^2
  Integrator : Integrator  InitialConditionSource=external
  Integrator1 : Integrator  InitialConditionSource=external
  Sum : Sum  Inputs=|+--
  U_filt : Outport
  U_DOT : Outport  Port=2
  wires:
  Integrator/1 -> [Y_DOT], Gain/1, Integrator1/1  "y_dot"
  Sum/1 -> Integrator/1  "y_dot_dot"
  Integrator1/1 -> Gain1/1, U_filt/1  "y"
  U/1 -> Gain2/1
  Gain2/1 -> Sum/1
  Gain/1 -> Sum/3
  Gain1/1 -> Sum/2
  [Y_DOT] -> U_DOT/1
  yD_0/1 -> Integrator/2
  y0/1 -> Integrator1/2

== system bh_COMPONENT_car_sys/Calc_LONG_LAT FORCES/Lateral_Tyre Force/Subsystem ==
  Fw_Y : Inport
  vB_mag : Inport  Port=2
  Constant : Constant  Value=0.005
  MATLAB Function : MATLAB Function  TreatAsAtomicUnit=on
  Fw_Yout : Outport
  wires:
  Constant/1 -> MATLAB Function/3(vel_thresh)
  vB_mag/1 -> MATLAB Function/2(vB_mag)
  Fw_Y/1 -> MATLAB Function/1(Fw_Y)
  MATLAB Function/1(Fw_Yout) -> Fw_Yout/1

== system bh_COMPONENT_car_sys/Calc_LONG_LAT FORCES/Lateral_Tyre Force/Subsystem1 ==
  Fw_Y : Inport
  vB_mag : Inport  Port=2
  Constant : Constant  Value=0.005
  MATLAB Function : MATLAB Function  TreatAsAtomicUnit=on
  Fw_Yout : Outport
  wires:
  Constant/1 -> MATLAB Function/3(vel_thresh)
  vB_mag/1 -> MATLAB Function/2(vB_mag)
  Fw_Y/1 -> MATLAB Function/1(Fw_Y)
  MATLAB Function/1(Fw_Yout) -> Fw_Yout/1

== system bh_COMPONENT_car_sys/Calc_LONG_LAT FORCES/Lateral_Tyre Force/Subsystem2 ==
  Fw_Y : Inport
  vB_mag : Inport  Port=2
  Constant : Constant  Value=0.005
  MATLAB Function : MATLAB Function  TreatAsAtomicUnit=on
  Fw_Yout : Outport
  wires:
  Constant/1 -> MATLAB Function/3(vel_thresh)
  vB_mag/1 -> MATLAB Function/2(vB_mag)
  Fw_Y/1 -> MATLAB Function/1(Fw_Y)
  MATLAB Function/1(Fw_Yout) -> Fw_Yout/1

== system bh_COMPONENT_car_sys/Calc_LONG_LAT FORCES/Lateral_Tyre Force/Subsystem3 ==
  Fw_Y : Inport
  vB_mag : Inport  Port=2
  Constant : Constant  Value=0.005
  MATLAB Function : MATLAB Function  TreatAsAtomicUnit=on
  Fw_Yout : Outport
  wires:
  Constant/1 -> MATLAB Function/3(vel_thresh)
  vB_mag/1 -> MATLAB Function/2(vB_mag)
  Fw_Y/1 -> MATLAB Function/1(Fw_Y)
  MATLAB Function/1(Fw_Yout) -> Fw_Yout/1

== system bh_COMPONENT_car_sys/Calc_LONG_LAT FORCES/Lateral_Tyre Force/corect_if_stationary ==
  f : TriggerPort  TriggerType=function-call  IsSimulinkFunction=on  FunctionName=correct_if_stationary  FunctionVisibility=scoped  VariantControl=(inherit)
  Constant : Constant  Value=0.005
  MATLAB Function : MATLAB Function  TreatAsAtomicUnit=on
  Fw_Y : ArgIn  DisableCoverage=on  ArgumentName=Fw_Y
  vb_MAG : ArgIn  DisableCoverage=on  Port=2  ArgumentName=vb_MAG
  y : ArgOut  DisableCoverage=on  ArgumentName=y
  wires:
  Fw_Y/1 -> MATLAB Function/1(Fw_Y)
  Constant/1 -> MATLAB Function/3(vel_thresh)
  vb_MAG/1 -> MATLAB Function/2(vB_mag)
  MATLAB Function/1(Fw_Yout) -> y/1

== system bh_COMPONENT_car_sys/Calc_LONG_LAT FORCES/Rolling_Resistance Force/Subsystem ==
  In1 : Inport
  1-D Lookup Table : Lookup_n-D  NumberOfTableDimensions=1  BreakpointsForDimension1=[0, 0.005, 0.01]  Table=[0,1,1]  ExtrapMethod=Clip  InternalRulePriority=Speed  RndMeth=Simplest  InputSameDT=on
  Abs : Abs
  Out1 : Outport
  wires:
  Abs/1 -> 1-D Lookup Table/1
  In1/1 -> Abs/1
  1-D Lookup Table/1 -> Out1/1

== system bh_COMPONENT_car_sys/Calc_LONG_LAT FORCES/Rolling_Resistance Force/Subsystem1 ==
  In1 : Inport
  1-D Lookup Table : Lookup_n-D  NumberOfTableDimensions=1  BreakpointsForDimension1=[0, 0.005, 0.01]  Table=[0,1,1]  ExtrapMethod=Clip  InternalRulePriority=Speed  RndMeth=Simplest  InputSameDT=on
  Abs : Abs
  Out1 : Outport
  wires:
  Abs/1 -> 1-D Lookup Table/1
  In1/1 -> Abs/1
  1-D Lookup Table/1 -> Out1/1

== system bh_COMPONENT_car_sys/Calc_LONG_LAT FORCES/Rolling_Resistance Force/Subsystem2 ==
  In1 : Inport
  1-D Lookup Table : Lookup_n-D  NumberOfTableDimensions=1  BreakpointsForDimension1=[0, 0.005, 0.01]  Table=[0,1,1]  ExtrapMethod=Clip  InternalRulePriority=Speed  RndMeth=Simplest  InputSameDT=on
  Abs : Abs
  Out1 : Outport
  wires:
  Abs/1 -> 1-D Lookup Table/1
  In1/1 -> Abs/1
  1-D Lookup Table/1 -> Out1/1

== system bh_COMPONENT_car_sys/Calc_LONG_LAT FORCES/Rolling_Resistance Force/Subsystem3 ==
  In1 : Inport
  1-D Lookup Table : Lookup_n-D  NumberOfTableDimensions=1  BreakpointsForDimension1=[0, 0.005, 0.01]  Table=[0,1,1]  ExtrapMethod=Clip  InternalRulePriority=Speed  RndMeth=Simplest  InputSameDT=on
  Abs : Abs
  Out1 : Outport
  wires:
  Abs/1 -> 1-D Lookup Table/1
  In1/1 -> Abs/1
  1-D Lookup Table/1 -> Out1/1

== system bh_COMPONENT_car_sys/Calc_LONG_LAT FORCES/Rolling_Resistance Force/do_0_to_1_for_velocity ==
  zero_to_1_from_VEL : TriggerPort  TriggerType=function-call  IsSimulinkFunction=on  FunctionName=zero_to_1_from_VEL  FunctionVisibility=scoped  VariantControl=(inherit)
  1-D Lookup Table : Lookup_n-D  NumberOfTableDimensions=1  BreakpointsForDimension1=[0, 0.005, 0.01]  Table=[0,1,1]  ExtrapMethod=Clip  InternalRulePriority=Speed  RndMeth=Simplest  InputSameDT=on
  Abs : Abs
  u : ArgIn  DisableCoverage=on  ArgumentName=u
  y : ArgOut  DisableCoverage=on  ArgumentName=y
  wires:
  Abs/1 -> 1-D Lookup Table/1
  1-D Lookup Table/1 -> y/1
  u/1 -> Abs/1

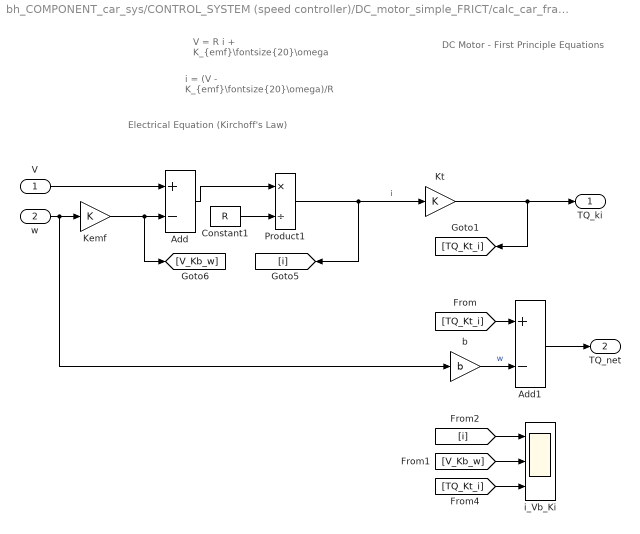
== system bh_COMPONENT_car_sys/CONTROL_SYSTEM (speed controller)/DC_motor_simple_FRICT/calc_car_frame_force/B1 ==
  note: Electrical Equation
      | (Kirchoff's Law)
  note: DC Motor - First Principle Equations
  note: V = R i + K_{emf}\fontsize{20}\omega
  note: i = (V - K_{emf}\fontsize{20}\omega)/R
  V : Inport
  w : Inport  Port=2
  Add : Sum  Inputs=+-
  Add1 : Sum  Inputs=+-
  Constant1 : Constant  Value=R
  Kemf : Gain  Gain=K
  Kt : Gain  Gain=K
  Product1 : Product  Inputs=*/
  b : Gain  Gain=b
  i_Vb_Ki : Scope  NumInputPorts=3
  TQ_ki : Outport
  TQ_net : Outport  Port=2
  wires:
  V/1 -> Add/1
  Product1/1 -> Kt/1, [i]  "i"
  Add/1 -> Product1/1
  Constant1/1 -> Product1/2
  w/1 -> b/1, Kemf/1
  Kemf/1 -> [V_Kb_w], Add/2
  Kt/1 -> TQ_ki/1, [TQ_Kt_i]
  [V_Kb_w] -> i_Vb_Ki/2
  [i] -> i_Vb_Ki/1
  [TQ_Kt_i] -> i_Vb_Ki/3
  [TQ_Kt_i] -> Add1/1
  b/1 -> Add1/2  "w"
  Add1/1 -> TQ_net/1

== system bh_COMPONENT_car_sys/CONTROL_SYSTEM (speed controller)/DC_motor_simple_FRICT/calc_car_frame_force/B3 ==
  note: V = R.(TQ / K) + K_{emf}\fontsize{20}\omega
  note: TQ = K.i
      | V = R i + K_{emf}\fontsize{20}\omega
  note: DC Motor - First Principle Equations
  note: Assuming SI: K=Kemf
  TQ : Inport
  w : Inport  Port=2
  Add : Sum
  Constant2 : Constant  Value=K
  Kemf : Gain  Gain=K
  Product2 : Product  Inputs=*/
  R : Gain  Gain=R
  V : Outport
  wires:
  R/1 -> Add/1
  Product2/1 -> R/1
  Constant2/1 -> Product2/2
  Kemf/1 -> Add/2
  w/1 -> Kemf/1
  Add/1 -> V/1
  TQ/1 -> Product2/1

== system bh_COMPONENT_car_sys/CONTROL_SYSTEM (speed controller)/DC_motor_simple_FRICT/calc_car_frame_force/calc_Ieqiv_axle ==
  Constant1 : Constant  Value=veh.shaft.I_common_rear_axle
  Constant5 : Constant  Value=mot_bR.J
  Constant7 : Constant  Value=veh.wheel.I
  Constant8 : Constant  Value=mot_bR.G
  Gain : Gain  Gain=2
  Math Function : Math  Operator=square  SaturateOnIntegerOverflow=on
  Product2 : Product
  Sum : Sum  Inputs=+|+
  Sum1 : Sum  Inputs=+|+
  I_equiv_axle : Outport
  wires:
  Constant7/1 -> Gain/1
  Constant8/1 -> Math Function/1
  Math Function/1 -> Product2/2  "G^2"
  Gain/1 -> Sum1/1
  Constant1/1 -> Sum1/2
  Constant5/1 -> Product2/1  "J1_motor"
  Product2/1 -> Sum/2
  Sum1/1 -> Sum/1  "J2_wheel_and_axle"
  Sum/1 -> I_equiv_axle/1

== system bh_COMPONENT_car_sys/CONTROL_SYSTEM (speed controller)/DC_motor_simple_FRICT/calc_car_frame_force/calc_beqiv_axle ==
  Constant5 : Constant  Value=mot_bR.B
  Constant7 : Constant  Value=veh.shaft.B
  Constant8 : Constant  Value=mot_bR.G
  Math Function : Math  Operator=square  SaturateOnIntegerOverflow=on
  Product2 : Product
  Sum : Sum  Inputs=+|+
  b_equiv_axle : Outport
  wires:
  Constant8/1 -> Math Function/1
  Math Function/1 -> Product2/2  "G^2"
  Constant5/1 -> Product2/1  "b1_motor"
  Product2/1 -> Sum/2  "b1_motor"
  Constant7/1 -> Sum/1  "b2_wheel_and_axle"
  Sum/1 -> b_equiv_axle/1

== system bh_COMPONENT_car_sys/CONTROL_SYSTEM (speed controller)/DC_motor_simple_FRICT/calc_car_frame_force/calc_mass_ONE_wheel ==
  note: Absorb HALF of the common axle mass
      | into each wheel
  Constant5 : Constant  Value=veh.shaft.m_common_rear_axle
  Constant7 : Constant  Value=veh.wheel.mass
  Gain : Gain  Gain=0.5
  Sum : Sum  Inputs=+|+
  m_ONE_wheel : Outport
  wires:
  Constant7/1 -> Sum/1
  Sum/1 -> m_ONE_wheel/1
  Constant5/1 -> Gain/1
  Gain/1 -> Sum/2

== system bh_COMPONENT_car_sys/CONTROL_SYSTEM (speed controller)/DC_motor_simple_FRICT/calc_car_frame_force/deriv_cal ==
  note: Y = U *     wn^2/( s^2 + 2*p*wn*s + wn^2)
      | Y*( s^2 + 2*p*wn*s + wn^2) = U * wn^2
      |
      | y'' + y'*2*p*wn + y*wn^2 = U*wn^2
  U : Inport
  y0 : Inport  Port=2
  yD_0 : Inport  Port=3
  Gain : Gain  Gain=2*p*wn
  Gain1 : Gain  Gain=wn^2
  Gain2 : Gain  Gain=wn^2
  Integrator : Integrator  InitialConditionSource=external
  Integrator1 : Integrator  InitialConditionSource=external
  Sum : Sum  Inputs=|+--
  U_filt : Outport
  U_DOT : Outport  Port=2
  wires:
  Integrator/1 -> [Y_DOT], Gain/1, Integrator1/1  "y_dot"
  Sum/1 -> Integrator/1  "y_dot_dot"
  Integrator1/1 -> Gain1/1, U_filt/1  "y"
  U/1 -> Gain2/1
  Gain2/1 -> Sum/1
  Gain/1 -> Sum/3
  Gain1/1 -> Sum/2
  [Y_DOT] -> U_DOT/1
  yD_0/1 -> Integrator/2
  y0/1 -> Integrator1/2

== matlab function bh_COMPONENT_car_sys/CONTROL_SYSTEM (speed controller)/DC_motor_simple_FRICT/calc_car_frame_force/MATLAB Function1 ==
  data: Tau_axle input; F_per_wheel output; theta_wheel_DD input; theta_wheel_D input; m_eq input; J_eq input; b_eq input; R input
function F_per_wheel = fcn(Tau_axle, theta_wheel_DD, theta_wheel_D, m_eq, J_eq, b_eq, R)

F_per_wheel = 0;


F_per_wheel = (    Tau_axle                             + ...
                -1 * theta_wheel_D  *  b_eq              + ...
                -1 * theta_wheel_DD * (J_eq + 2*m_eq*R^2)  ...
               ) / (2*R);

== matlab function bh_COMPONENT_car_sys/CONTROL_SYSTEM (speed controller)/DC_motor_simple_FRICT/calc_car_frame_force/MATLAB Function ==
  data: F_wheel input; tau_axle output; theta_wheel_DD input; theta_wheel_D input; m_eq input; J_eq input; b_eq input; R input
function tau_axle = fcn(F_wheel, theta_wheel_DD, theta_wheel_D, m_eq, J_eq, b_eq, R)

tau_axle = 0;

% T_axle = G * T_motor

tau_axle =  2*R*F_wheel                          + ...
            theta_wheel_DD * (J_eq + 2*m_eq*R^2) + ...
            theta_wheel_D  *  b_eq;

== matlab function bh_COMPONENT_car_sys/Calc_LONG_LAT FORCES/Lateral_Tyre Force/Subsystem/MATLAB Function ==
  data: Fw_Y input; vB_mag input; vel_thresh input; Fw_Yout output
function Fw_Yout = fcn(Fw_Y, vB_mag, vel_thresh)

if(vB_mag <= vel_thresh)

     Fw_Yout =  0;
else
     Fw_Yout =  Fw_Y; 
end

== matlab function bh_COMPONENT_car_sys/Calc_LONG_LAT FORCES/Lateral_Tyre Force/corect_if_stationary/MATLAB Function ==
  data: Fw_Y input; vB_mag input; vel_thresh input; Fw_Yout output
function Fw_Yout = fcn(Fw_Y, vB_mag, vel_thresh)

if(vB_mag <= vel_thresh)

     Fw_Yout =  0;
else
     Fw_Yout =  Fw_Y; 
end

== matlab function bh_COMPONENT_car_sys/Calc_LONG_LAT FORCES/Lateral_Tyre Force/Subsystem1/MATLAB Function ==
  data: Fw_Y input; vB_mag input; vel_thresh input; Fw_Yout output
function Fw_Yout = fcn(Fw_Y, vB_mag, vel_thresh)

if(vB_mag <= vel_thresh)

     Fw_Yout =  0;
else
     Fw_Yout =  Fw_Y; 
end

== matlab function bh_COMPONENT_car_sys/Calc_LONG_LAT FORCES/Lateral_Tyre Force/Subsystem2/MATLAB Function ==
  data: Fw_Y input; vB_mag input; vel_thresh input; Fw_Yout output
function Fw_Yout = fcn(Fw_Y, vB_mag, vel_thresh)

if(vB_mag <= vel_thresh)

     Fw_Yout =  0;
else
     Fw_Yout =  Fw_Y; 
end

== matlab function bh_COMPONENT_car_sys/Calc_LONG_LAT FORCES/Lateral_Tyre Force/Subsystem3/MATLAB Function ==
  data: Fw_Y input; vB_mag input; vel_thresh input; Fw_Yout output
function Fw_Yout = fcn(Fw_Y, vB_mag, vel_thresh)

if(vB_mag <= vel_thresh)

     Fw_Yout =  0;
else
     Fw_Yout =  Fw_Y; 
end
